simulink model "newtrajexperiment"  (R2016a)
settings: Solver=ode5  StartTime=0.0  StopTime=inf  FixedStep=0.001  RelTol=1e-3
libraries: dcpctrl x1
settings Model: SimulationMode=external  Creator=julianleland  LastModifiedBy=julianleland
settings HardwareCC: ProdBitPerLong=64  ProdLargestAtomicFloat=None  ProdHWDeviceType=Intel->x86-64  TargetBitPerLong=64  TargetBitPerPointer=64  TargetIntDivRoundTo=Zero  TargetEndianess=LittleEndian  TargetWordSize=64  TargetHWDeviceType=Intel->x86-64
settings RTWCC: SystemTargetFile=sldrt.tlc  TemplateMakefile=sldrt.tmf  Description=Simulink Desktop Real-Time  RTWCompilerOptimization=on
settings CodeAppCC: MaxIdLength=95
settings SimulinkDesktopRealTimeCC: TargetPreCompLibLocation=/Applications/MATLAB_R2016a.app/toolbox/sldrt/lib/maci64  TargetLangStandard=C89/C90 (ANSI)  SupportVariableSizeSignals=off

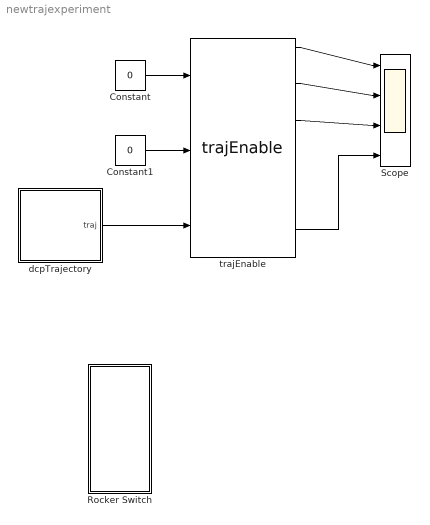
== system newtrajexperiment ==
  Constant : Constant  Value=0
  Constant1 : Constant  Value=0
  Rocker Switch : Subsystem  DialogController=hmiCreateDDGDialog  IsWebBlock=on  mask(MWDashboardBlock){webBlockId=8c2d6718-217a-4a37-a815-c2a64da9dba8, webBlockType=rockerswitch, ShowInLibBrowser=on, ShowInitialText=on, HMISrcModelName=newtrajexperiment}
      mask prompts: webBlockId "WebBlock Id"; webBlockType "WebBlock Type"; HMISrcModelName "Source Model"
      mask Help: helpview([docroot '/mapfiles/simulink.map'], 'hmi_rocker_switch')
      mask Display:
      | if strcmp(get_param(bdroot(gcb),'BlockDiagramType'), 'library')
      |     image([(matlabroot) '/toolbox/simulink/hmi/icons/RockerSwitch.png']);
      | end
  Scope : Scope  NumInputPorts=4
  dcpTrajectory : Subsystem
  trajEnable : dcpctrl/trajEnable
  wires:
  dcpTrajectory/1(traj) -> trajEnable/3
  Constant/1 -> trajEnable/1
  trajEnable/1 -> Scope/1
  trajEnable/3 -> Scope/2
  trajEnable/5 -> Scope/3
  trajEnable/11 -> Scope/4
  Constant1/1 -> trajEnable/2

== system newtrajexperiment/Rocker Switch ==

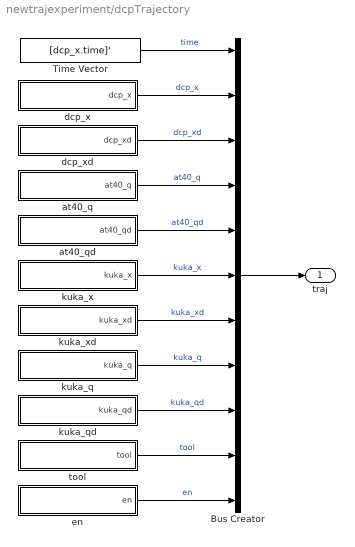
== system newtrajexperiment/dcpTrajectory ==
  Bus Creator : BusCreator  Inputs=11
  Time Vector : FromWorkspace  VariableName=[dcp_x.time]'  SampleTime=0
  at40_q : Subsystem
  at40_qd : Subsystem
  dcp_x : Subsystem
  dcp_xd : Subsystem
  en : Subsystem
  kuka_q : Subsystem
  kuka_qd : Subsystem
  kuka_x : Subsystem
  kuka_xd : Subsystem
  tool : Subsystem
  traj : Outport
  wires:
  Bus Creator/1 -> traj/1
  at40_qd/1(at40_qd) -> Bus Creator/5  "at40_qd"
  dcp_xd/1(dcp_xd) -> Bus Creator/3  "dcp_xd"
  Time Vector/1 -> Bus Creator/1  "time"
  at40_q/1(at40_q) -> Bus Creator/4  "at40_q"
  kuka_x/1(kuka_x) -> Bus Creator/6  "kuka_x"
  kuka_xd/1(kuka_xd) -> Bus Creator/7  "kuka_xd"
  kuka_q/1(kuka_q) -> Bus Creator/8  "kuka_q"
  kuka_qd/1(kuka_qd) -> Bus Creator/9  "kuka_qd"
  tool/1(tool) -> Bus Creator/10  "tool"
  en/1(en) -> Bus Creator/11  "en"
  dcp_x/1(dcp_x) -> Bus Creator/2  "dcp_x"

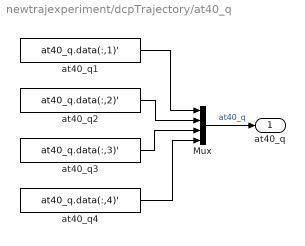
== system newtrajexperiment/dcpTrajectory/at40_q ==
  Mux : Mux
  at40_q1 : FromWorkspace  VariableName=at40_q.data(:,1)'  SampleTime=0
  at40_q2 : FromWorkspace  VariableName=at40_q.data(:,2)'  SampleTime=0
  at40_q3 : FromWorkspace  VariableName=at40_q.data(:,3)'  SampleTime=0
  at40_q4 : FromWorkspace  VariableName=at40_q.data(:,4)'  SampleTime=0
  at40_q : Outport
  wires:
  Mux/1 -> at40_q/1  "at40_q"
  at40_q2/1 -> Mux/2
  at40_q1/1 -> Mux/1
  at40_q3/1 -> Mux/3
  at40_q4/1 -> Mux/4

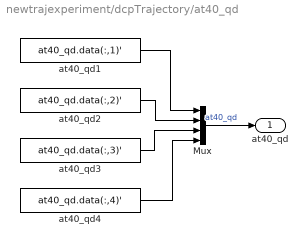
== system newtrajexperiment/dcpTrajectory/at40_qd ==
  Mux : Mux
  at40_qd1 : FromWorkspace  VariableName=at40_qd.data(:,1)'  SampleTime=0
  at40_qd2 : FromWorkspace  VariableName=at40_qd.data(:,2)'  SampleTime=0
  at40_qd3 : FromWorkspace  VariableName=at40_qd.data(:,3)'  SampleTime=0
  at40_qd4 : FromWorkspace  VariableName=at40_qd.data(:,4)'  SampleTime=0
  at40_qd : Outport
  wires:
  Mux/1 -> at40_qd/1  "at40_qd"
  at40_qd2/1 -> Mux/2
  at40_qd1/1 -> Mux/1
  at40_qd3/1 -> Mux/3
  at40_qd4/1 -> Mux/4

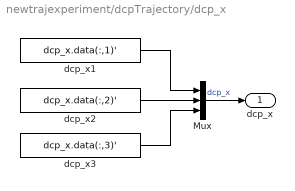
== system newtrajexperiment/dcpTrajectory/dcp_x ==
  Mux : Mux  Inputs=3
  dcp_x1 : FromWorkspace  VariableName=dcp_x.data(:,1)'  SampleTime=0
  dcp_x2 : FromWorkspace  VariableName=dcp_x.data(:,2)'  SampleTime=0
  dcp_x3 : FromWorkspace  VariableName=dcp_x.data(:,3)'  SampleTime=0
  dcp_x : Outport
  wires:
  Mux/1 -> dcp_x/1  "dcp_x"
  dcp_x2/1 -> Mux/2
  dcp_x1/1 -> Mux/1
  dcp_x3/1 -> Mux/3

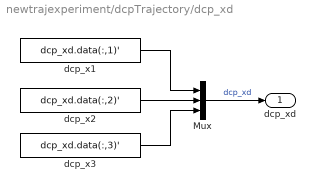
== system newtrajexperiment/dcpTrajectory/dcp_xd ==
  Mux : Mux  Inputs=3
  dcp_x1 : FromWorkspace  VariableName=dcp_xd.data(:,1)'  SampleTime=0
  dcp_x2 : FromWorkspace  VariableName=dcp_xd.data(:,2)'  SampleTime=0
  dcp_x3 : FromWorkspace  VariableName=dcp_xd.data(:,3)'  SampleTime=0
  dcp_xd : Outport
  wires:
  Mux/1 -> dcp_xd/1  "dcp_xd"
  dcp_x2/1 -> Mux/2
  dcp_x1/1 -> Mux/1
  dcp_x3/1 -> Mux/3

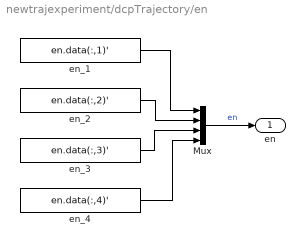
== system newtrajexperiment/dcpTrajectory/en ==
  Mux : Mux
  en_1 : FromWorkspace  VariableName=en.data(:,1)'  SampleTime=0
  en_2 : FromWorkspace  VariableName=en.data(:,2)'  SampleTime=0
  en_3 : FromWorkspace  VariableName=en.data(:,3)'  SampleTime=0
  en_4 : FromWorkspace  VariableName=en.data(:,4)'  SampleTime=0
  en : Outport
  wires:
  Mux/1 -> en/1  "en"
  en_2/1 -> Mux/2
  en_1/1 -> Mux/1
  en_3/1 -> Mux/3
  en_4/1 -> Mux/4

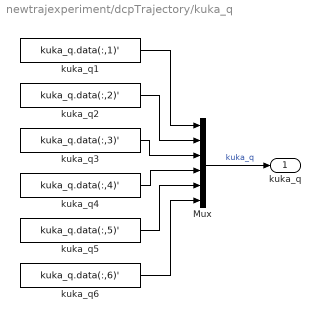
== system newtrajexperiment/dcpTrajectory/kuka_q ==
  Mux : Mux  Inputs=6
  kuka_q1 : FromWorkspace  VariableName=kuka_q.data(:,1)'  SampleTime=0
  kuka_q2 : FromWorkspace  VariableName=kuka_q.data(:,2)'  SampleTime=0
  kuka_q3 : FromWorkspace  VariableName=kuka_q.data(:,3)'  SampleTime=0
  kuka_q4 : FromWorkspace  VariableName=kuka_q.data(:,4)'  SampleTime=0
  kuka_q5 : FromWorkspace  VariableName=kuka_q.data(:,5)'  SampleTime=0
  kuka_q6 : FromWorkspace  VariableName=kuka_q.data(:,6)'  SampleTime=0
  kuka_q : Outport
  wires:
  Mux/1 -> kuka_q/1  "kuka_q"
  kuka_q2/1 -> Mux/2
  kuka_q1/1 -> Mux/1
  kuka_q3/1 -> Mux/3
  kuka_q4/1 -> Mux/4
  kuka_q5/1 -> Mux/5
  kuka_q6/1 -> Mux/6

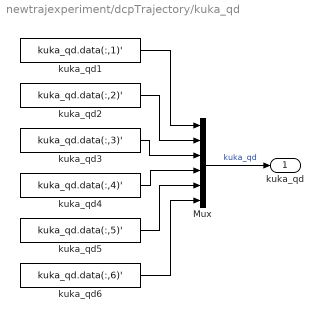
== system newtrajexperiment/dcpTrajectory/kuka_qd ==
  Mux : Mux  Inputs=6
  kuka_qd1 : FromWorkspace  VariableName=kuka_qd.data(:,1)'  SampleTime=0
  kuka_qd2 : FromWorkspace  VariableName=kuka_qd.data(:,2)'  SampleTime=0
  kuka_qd3 : FromWorkspace  VariableName=kuka_qd.data(:,3)'  SampleTime=0
  kuka_qd4 : FromWorkspace  VariableName=kuka_qd.data(:,4)'  SampleTime=0
  kuka_qd5 : FromWorkspace  VariableName=kuka_qd.data(:,5)'  SampleTime=0
  kuka_qd6 : FromWorkspace  VariableName=kuka_qd.data(:,6)'  SampleTime=0
  kuka_qd : Outport
  wires:
  Mux/1 -> kuka_qd/1  "kuka_qd"
  kuka_qd2/1 -> Mux/2
  kuka_qd1/1 -> Mux/1
  kuka_qd3/1 -> Mux/3
  kuka_qd4/1 -> Mux/4
  kuka_qd5/1 -> Mux/5
  kuka_qd6/1 -> Mux/6

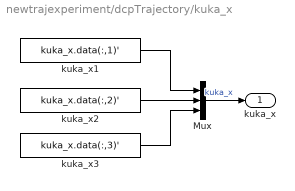
== system newtrajexperiment/dcpTrajectory/kuka_x ==
  Mux : Mux  Inputs=3
  kuka_x1 : FromWorkspace  VariableName=kuka_x.data(:,1)'  SampleTime=0
  kuka_x2 : FromWorkspace  VariableName=kuka_x.data(:,2)'  SampleTime=0
  kuka_x3 : FromWorkspace  VariableName=kuka_x.data(:,3)'  SampleTime=0
  kuka_x : Outport
  wires:
  Mux/1 -> kuka_x/1  "kuka_x"
  kuka_x2/1 -> Mux/2
  kuka_x1/1 -> Mux/1
  kuka_x3/1 -> Mux/3

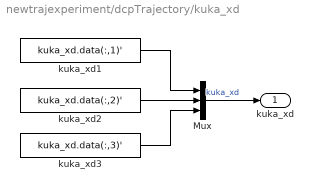
== system newtrajexperiment/dcpTrajectory/kuka_xd ==
  Mux : Mux  Inputs=3
  kuka_xd1 : FromWorkspace  VariableName=kuka_xd.data(:,1)'  SampleTime=0
  kuka_xd2 : FromWorkspace  VariableName=kuka_xd.data(:,2)'  SampleTime=0
  kuka_xd3 : FromWorkspace  VariableName=kuka_xd.data(:,3)'  SampleTime=0
  kuka_xd : Outport
  wires:
  Mux/1 -> kuka_xd/1  "kuka_xd"
  kuka_xd2/1 -> Mux/2
  kuka_xd1/1 -> Mux/1
  kuka_xd3/1 -> Mux/3

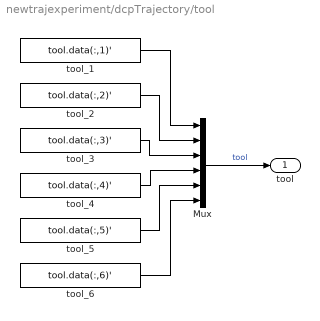
== system newtrajexperiment/dcpTrajectory/tool ==
  Mux : Mux  Inputs=6
  tool_1 : FromWorkspace  VariableName=tool.data(:,1)'  SampleTime=0
  tool_2 : FromWorkspace  VariableName=tool.data(:,2)'  SampleTime=0
  tool_3 : FromWorkspace  VariableName=tool.data(:,3)'  SampleTime=0
  tool_4 : FromWorkspace  VariableName=tool.data(:,4)'  SampleTime=0
  tool_5 : FromWorkspace  VariableName=tool.data(:,5)'  SampleTime=0
  tool_6 : FromWorkspace  VariableName=tool.data(:,6)'  SampleTime=0
  tool : Outport
  wires:
  Mux/1 -> tool/1  "tool"
  tool_2/1 -> Mux/2
  tool_1/1 -> Mux/1
  tool_3/1 -> Mux/3
  tool_4/1 -> Mux/4
  tool_5/1 -> Mux/5
  tool_6/1 -> Mux/6
